simulink model "model_FS_PSH_IEEE39"  (R2020b)
settings: Solver=ode3  StartTime=0.0  StopTime=300  FixedStep=Ts  RelTol=1e-3
PostLoadFcn:
  | IEEE39BusLineLength;
  | vNomHV = 345E3;fNom=60;load('Dynamicload.mat');
InitFcn:
  | IEEE39BusLineLength;
  | vNomHV = 345E3;fNom=60;load('Dynamicload.mat');
values from neighbouring files (symbols this model uses):
  Rp = 0.05    [IEEE39BusLineLength.m]
  t_sw_off = 220    [MAIN_FS_PSH_IEEE39.m]    (also in MAIN_T_PSH_IEEE39.m; MAIN_VS_PSH.m = 45)
  t_sw_on = 130    [MAIN_FS_PSH_IEEE39.m]    (also in MAIN_T_PSH_IEEE39.m; MAIN_VS_PSH.m = 35)
  TL_10_11_len = 14    [IEEE39BusLineLength.m]
  TL_10_13_len = 14    [IEEE39BusLineLength.m]
  TL_13_14_len = 32    [IEEE39BusLineLength.m]
  TL_14_15_len = 70    [IEEE39BusLineLength.m]
  TL_15_16_len = 31.5    [IEEE39BusLineLength.m]
  TL_16_17_len = 26    [IEEE39BusLineLength.m]
  TL_16_19_len = 61    [IEEE39BusLineLength.m]
  TL_16_21_len = 46    [IEEE39BusLineLength.m]
  TL_16_24_len = 15    [IEEE39BusLineLength.m]
  TL_17_18_len = 26    [IEEE39BusLineLength.m]
  TL_17_27_len = 59    [IEEE39BusLineLength.m]
  TL_1_2_len = 134    [IEEE39BusLineLength.m]
  TL_1_39_len = 105    [IEEE39BusLineLength.m]
  TL_21_22_len = 47    [IEEE39BusLineLength.m]
  TL_22_23_len = 33    [IEEE39BusLineLength.m]
  TL_24_23_len = 88    [IEEE39BusLineLength.m]
  TL_25_26_len = 101    [IEEE39BusLineLength.m]
  TL_26_27_len = 46.5    [IEEE39BusLineLength.m]
  TL_26_28_len = 151    [IEEE39BusLineLength.m]
  TL_26_29_len = 200    [IEEE39BusLineLength.m]
  TL_28_29_len = 48    [IEEE39BusLineLength.m]
  TL_2_25_len = 28    [IEEE39BusLineLength.m]
  TL_2_2_len = 49    [IEEE39BusLineLength.m]
  TL_3_18_len = 42    [IEEE39BusLineLength.m]
  TL_3_4_len = 53    [IEEE39BusLineLength.m]
  TL_4_14_len = 33    [IEEE39BusLineLength.m]
  TL_4_5_len = 32.5    [IEEE39BusLineLength.m]
  TL_5_6_len = 14    [IEEE39BusLineLength.m]
  TL_5_8_len = 32    [IEEE39BusLineLength.m]
  TL_6_11_len = 26.5    [IEEE39BusLineLength.m]
  TL_6_7_len = 25.5    [IEEE39BusLineLength.m]
  TL_7_8_len = 15    [IEEE39BusLineLength.m]
  TL_8_9_len = 93    [IEEE39BusLineLength.m]
  TL_9_39_len = 136    [IEEE39BusLineLength.m]
  Ts = 25e-6    (= 2.5e-05)    [MAIN_FS_PSH_IEEE39.m]    (also in MAIN_T_PSH_IEEE39.m; MAIN_VS_PSH.m = 1e-07)
undefined symbols (not defined in the file or in its folder): D1, Delta, FS_PSH, load15, load16, load18, load20, load21, load23, load24, load25, load26, load27, load28, load29, load3, load39, load4, load7, load8
libraries: powerlib x216, sps_avr x10, powerlib_meascontrol x5, pid_lib x1
(part 5 of 8)

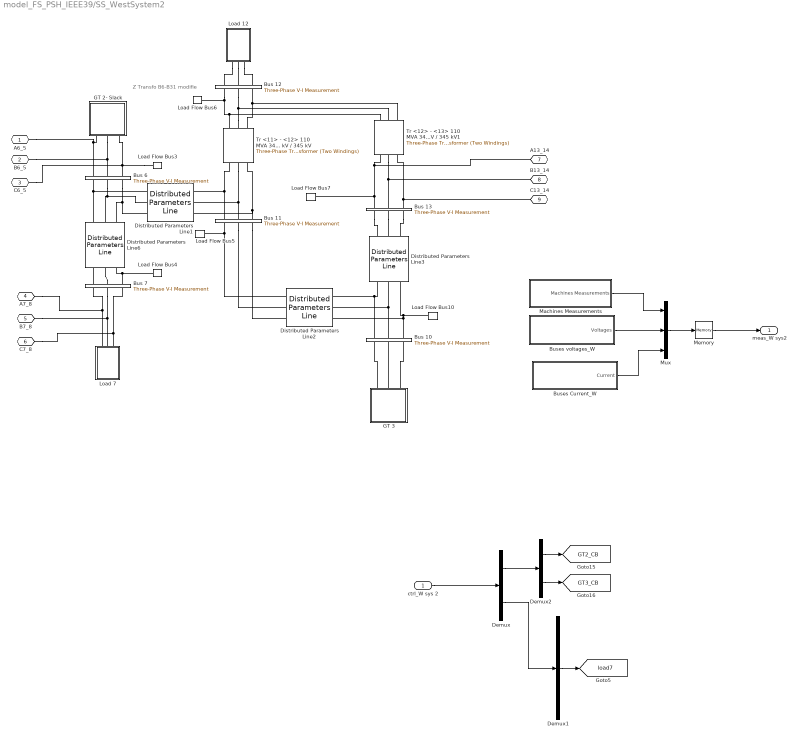
== system model_FS_PSH_IEEE39/SS_WestSystem2 ==
  note: Z Transfo B6-B31 modifie
  ctrl_W sys 2 : Inport
  Bus 10 : powerlib/Measurements/Three-Phase V-I Measurement  VoltageMeasurement=phase-to-ground  SetLabelV=on  LabelV=V_bus_10  Vpu=off  VpuLL=off  CurrentMeasurement=yes  SetLabelI=on  LabelI=I_bus_10  Ipu=off  Pbase=100e6  Vbase=230e3  OutputType=Complex  PhasorSimulation=off  PSBequivalent=0
  Bus 11 : powerlib/Measurements/Three-Phase V-I Measurement  VoltageMeasurement=phase-to-ground  SetLabelV=on  LabelV=V_bus_11  Vpu=off  VpuLL=off  CurrentMeasurement=yes  SetLabelI=on  LabelI=I_bus_11  Ipu=off  Pbase=100e6  Vbase=230e3  OutputType=Complex  PhasorSimulation=off  PSBequivalent=0
  Bus 12 : powerlib/Measurements/Three-Phase V-I Measurement  VoltageMeasurement=phase-to-ground  SetLabelV=on  LabelV=V_bus_12  Vpu=off  VpuLL=off  CurrentMeasurement=yes  SetLabelI=on  LabelI=I_bus_12  Ipu=off  Pbase=100e6  Vbase=230e3  OutputType=Complex  PhasorSimulation=off  PSBequivalent=0
  Bus 13 : powerlib/Measurements/Three-Phase V-I Measurement  VoltageMeasurement=phase-to-ground  SetLabelV=on  LabelV=V_bus_13  Vpu=off  VpuLL=off  CurrentMeasurement=yes  SetLabelI=on  LabelI=I_bus_13  Ipu=off  Pbase=100e6  Vbase=230e3  OutputType=Complex  PhasorSimulation=off  PSBequivalent=0
  Bus 6 : powerlib/Measurements/Three-Phase V-I Measurement  VoltageMeasurement=phase-to-ground  SetLabelV=on  LabelV=V_bus_6  Vpu=off  VpuLL=off  CurrentMeasurement=yes  SetLabelI=on  LabelI=I_bus_6  Ipu=off  Pbase=100e6  Vbase=230e3  OutputType=Complex  PhasorSimulation=off  PSBequivalent=0
  Bus 7 : powerlib/Measurements/Three-Phase V-I Measurement  VoltageMeasurement=phase-to-ground  SetLabelV=on  LabelV=V_bus_7  Vpu=off  VpuLL=off  CurrentMeasurement=yes  SetLabelI=on  LabelI=I_bus_7  Ipu=off  Pbase=100e6  Vbase=230e3  OutputType=Complex  PhasorSimulation=off  PSBequivalent=0
  Buses Current_W : Subsystem
  Buses voltages_W : Subsystem
  Demux : Demux  Outputs=[2 2]
  Demux1 : Demux  Outputs=[2 ]
  Demux2 : Demux  Outputs=2
  Distributed Parameters Line1 : powerlib/Elements/Distributed Parameters Line  Phases=3  Length=TL_6_11_len  Frequency=fNom  Resistance=[0.833 3.333]/TL_6_11_len  Inductance="[0.026  0.078]/TL_6_11_len"  Capacitance=[0.31e-6 0.141e-6]/TL_6_11_len  x1=[-0.000125 4.90236813149437e-09 0 0;-0.0001 4.73761402312569e-09 183127.021005182 -193527.239892428;-7.5e-05 4.57243909248611e-09 184942.800795633 -191792.737027805;-5e-05 4.40685801136803e-09 186742.152897159 -190041.198023314;-2.5e-05 4.2408854876405e-09 188524.917480904 -188272.778460778]  x2=[-0.000125 -1.4342554633322e-08 0 0;-0.0001 -1.44743326982834e-08 188556.811701446 -190108.544883478;-7.5e-05 -1.46048250693224e-08 190340.130987805 -188323.021034435;-5e-05 -1.47340201553523e-08 192106.543163165 -186520.769245761;-2.5e-05 -1.48619064805184e-08 193855.891324581 -184701.949603881]  x3=[-0.000125 -1.81011006279439e-10 0 0;-0.0001 -1.87198811943795e-10 1012.19433406295 -1197.40014896563;-7.5e-05 -1.93369989527271e-10 1023.43451008816 -1187.80734434082;-5e-05 -1.99523990870192e-10 1034.58377874259 -1178.10903179967;-2.5e-05 -2.05660269338577e-10 1045.64114968372 -1168.30607280236]  x4=[-0.000125 1.68385779335451e-10 0 0;-0.0001 1.74132809904858e-10 246.070217535326 -146.122053826147;-7.5e-05 1.79864372991236e-10 247.436293615228 -143.796492599063;-5e-05 1.85579959484012e-10 248.780390972829 -141.45815853606;-2.5e-05 1.91279061691744e-10 250.102390217632 -139.107259341491]  x5=0.000104871349757691  V1=ones(3,3)  V2=ones(3,3)  I1=ones(3,3)  I2=ones(3,3)  nHarmo=1  Measurements=None  Decoupling=off  VsMag0=0  VrMag0=0  VsAngle0=0  VrAngle0=0  IsMag0=0  IrMag0=0  IsAngle0=0  IrAngle0=0
  Distributed Parameters Line2 : powerlib/Elements/Distributed Parameters Line  Phases=3  Length=TL_10_11_len  Frequency=fNom  Resistance=[0.476 1.904]/TL_10_11_len  Inductance="[0.014  0.04]/TL_10_11_len"  Capacitance=[0.162e-6 0.074e-6]/TL_10_11_len  x1=[-7.5e-05 -1.46049279170452e-08 0 0;-5e-05 -1.47340887255765e-08 192106.543163165 -186520.769245761;-2.5e-05 -1.48619407671533e-08 193855.891324581 -184701.949603881]  x2=[-7.5e-05 -2.31631319093915e-08 0 0;-5e-05 -2.32876424160693e-08 195466.101592622 -184887.987151561;-2.5e-05 -2.34100843796963e-08 197199.912483554 -183037.577926856]  x3=[-7.5e-05 -1.20973818921581e-10 0 0;-5e-05 -1.26341409378821e-10 1010.52803842152 -1242.83594676881;-2.5e-05 -1.31697777461561e-10 1022.19650500434 -1233.25683348948]  x4=[-7.5e-05 7.40590073052612e-11 0 0;-5e-05 7.90894066759697e-11 294.937649217573 -30.8703627073713;-2.5e-05 8.41127808682744e-11 295.215353287942 -28.08936050336]  x5=5.44058820349418e-05  V1=ones(3,3)  V2=ones(3,3)  I1=ones(3,3)  I2=ones(3,3)  nHarmo=1  Measurements=None  Decoupling=off  VsMag0=0  VrMag0=0  VsAngle0=0  VrAngle0=0  IsMag0=0  IrMag0=0  IsAngle0=0  IrAngle0=0
  Distributed Parameters Line3 : powerlib/Elements/Distributed Parameters Line  Phases=3  Length=TL_10_13_len  Frequency=fNom  Resistance=[0.476 1.904]/TL_10_13_len  Inductance=[0.014 0.04]/TL_10_13_len  Capacitance=[0.162e-6 0.074e-6]/TL_10_13_len  x1=[-7.5e-05 -1.85919269091365e-08 0 0;-5e-05 -1.87360708053477e-08 257967.853677424 -71921.0706051768;-2.5e-05 -1.88785504554162e-08 257278.56069942 -74349.1214410131]  x2=[-7.5e-05 -2.31631319093915e-08 0 0;-5e-05 -2.32876424160693e-08 257850.744524134 -76834.6159821403;-2.5e-05 -2.34100843796963e-08 257115.148573608 -79261.3448713978]  x3=[-7.5e-05 -1.9729013706856e-10 0 0;-5e-05 -2.00122610987713e-10 1799.42783654337 -341.693872198189;-2.5e-05 -2.02937308859429e-10 1796.12756372396 -358.637663817273]  x4=[-7.5e-05 1.41714968743232e-10 0 0;-5e-05 1.44134764486409e-10 -42.3684337823979 -147.97249719393;-2.5e-05 1.46541757346403e-10 -43.7611636427956 -147.566548222069]  x5=5.44058820349418e-05  V1=ones(3,3)  V2=ones(3,3)  I1=ones(3,3)  I2=ones(3,3)  nHarmo=1  Measurements=None  Decoupling=off  VsMag0=0  VrMag0=0  VsAngle0=0  VrAngle0=0  IsMag0=0  IrMag0=0  IsAngle0=0  IrAngle0=0
  Distributed Parameters Line6 : powerlib/Elements/Distributed Parameters Line  Phases=3  Length=TL_6_7_len  Frequency=fNom  Resistance=[0.714 2.857]/TL_6_7_len  Inductance=[0.029 0.087]/TL_6_7_len  Capacitance=[0.252e-6 0.114e-6]/TL_6_7_len  x1=[-0.0001 4.73761402312569e-09 259163.016573719 -61829.0323636399;-7.5e-05 4.57243909248611e-09 258568.782925244 -64268.7952221604;-5e-05 4.40685801136803e-09 257951.581702399 -66702.8493546806;-2.5e-05 4.2408854876405e-09 257311.467728565 -69130.9785544385]  x2=[-0.0001 4.12646376630165e-09 259289.948818673 -48646.1844692721;-7.5e-05 3.96483863419745e-09 258819.953112779 -51087.7289997077;-5e-05 3.80286132220067e-09 258326.967522127 -53524.7356226591;-2.5e-05 3.64054621807272e-09 257811.035836546 -55956.9878691072]  x3=[-0.0001 -8.28425316453442e-12 -433.188488031618 -79.7957266342144;-7.5e-05 -8.62804148707643e-12 -433.921305740028 -75.7095112058845;-5e-05 -8.97106341708535e-12 -434.615580049085 -71.6165708210094;-2.5e-05 -9.31328848536999e-12 -435.271249289331 -67.5172690382197]  x4=[-0.0001 1.51239119220935e-11 1964.32766038478 -220.748781181744;-7.5e-05 1.5097572753948e-11 1962.15991096584 -239.252028488418;-5e-05 1.50698925320947e-11 1959.8178711582 -257.734024046541;-2.5e-05 1.50408737152511e-11 1957.30174899538 -276.193126178405]  x5=9.9589156036187e-05  V1=ones(3,3)  V2=ones(3,3)  I1=ones(3,3)  I2=ones(3,3)  nHarmo=1  Measurements=None  Decoupling=off  VsMag0=0  VrMag0=0  VsAngle0=0  VrAngle0=0  IsMag0=0  IrMag0=0  IsAngle0=0  IrAngle0=0
  GT 2- Slack : Subsystem
  GT 3 : Subsystem
  Load 12 : Subsystem
  Load 7 : Subsystem
  Load Flow Bus10 : powerlib/Measurements/Load Flow Bus  LConnTagsString=a  Phases=single  Connectors=on one side  ID=Bus-10  Vbase=345e+003  Vref=1  Vangle=0  VLF=1.011  VLFb=1  VLFc=1  angleLF=22.22  angleLFb=0  angleLFc=0
      settings: AttributesFormatString=%<ID>\n%<Vbase>V\n%<VLF>pu\n%<angleLF>deg.
  Load Flow Bus3 : powerlib/Measurements/Load Flow Bus  LConnTagsString=a  Phases=single  Connectors=on one side  ID=Bus-6  Vbase=345e+003  Vref=1  Vangle=0  VLF=1.003  VLFb=1  VLFc=1  angleLF=20.92  angleLFb=0  angleLFc=0
      settings: AttributesFormatString=%<ID>\n%<Vbase>V\n%<VLF>pu\n%<angleLF>deg.
  Load Flow Bus4 : powerlib/Measurements/Load Flow Bus  LConnTagsString=a  Phases=single  Connectors=on one side  ID=Bus-7  Vbase=345e+003  Vref=1  Vangle=0  VLF=0.9928  VLFb=1  VLFc=1  angleLF=19.19  angleLFb=0  angleLFc=0
      settings: AttributesFormatString=%<ID>\n%<Vbase>V\n%<VLF>pu\n%<angleLF>deg.
  Load Flow Bus5 : powerlib/Measurements/Load Flow Bus  LConnTagsString=a  Phases=single  Connectors=on one side  ID=Bus-11  Vbase=345e+003  Vref=1  Vangle=0  VLF=1.007  VLFb=1  VLFc=1  angleLF=21.76  angleLFb=0  angleLFc=0
      settings: AttributesFormatString=%<ID>\n%<Vbase>V\n%<VLF>pu\n%<angleLF>deg.
  Load Flow Bus6 : powerlib/Measurements/Load Flow Bus  LConnTagsString=a  Phases=single  Connectors=on one side  ID=Bus-12  Vbase=345e+003  Vref=1  Vangle=0  VLF=0.996  VLFb=1  VLFc=1  angleLF=51.6  angleLFb=0  angleLFc=0
      settings: AttributesFormatString=%<ID>\n%<Vbase>V\n%<VLF>pu\n%<angleLF>deg.
  Load Flow Bus7 : powerlib/Measurements/Load Flow Bus  LConnTagsString=a  Phases=single  Connectors=on one side  ID=Bus-13  Vbase=345e+003  Vref=1  Vangle=0  VLF=1.007  VLFb=1  VLFc=1  angleLF=21.59  angleLFb=0  angleLFc=0
      settings: AttributesFormatString=%<ID>\n%<Vbase>V\n%<VLF>pu\n%<angleLF>deg.
  Machines Measurements : Subsystem
      mask Display: disp('Machines Measurements')
  Memory : Memory
  Mux : Mux  Inputs=3
  Tr <11> - <12> 110 MVA 345 kV / 345 kV : powerlib/Elements/Three-Phase Transformer (Two Windings)  Winding1Connection=Delta (D1)  Winding2Connection=Yg  CoreType=Three single-phase transformers  SetSaturation=off  Hysteresis=off  DataFile='hysteresis'  SetInitialFlux=off  Measurements=None  UNITS=pu  NominalPower=[ 110e6 fNom]  Winding1="[345e3 0.0016*110/100/2   0.0435*110/100/2]"  Winding2="[ 1.006*345e3 0.0016*110/100/2   0.0435*110/100/2]"  Rm=500  Lm=500  L0=0.5  Saturation="[ 0,0  ;  0.005,1.2  ;  1.0,1.4 ]"  InitialFluxes=[ 0.8 , -0.8 , 0.7 ]  BreakLoop=off  DiscreteSolver=Trapezoidal iterative  DataType=off  TransfoNumber=0
  Tr <12> - <13> 110 MVA 345 kV / 345 kV1 : powerlib/Elements/Three-Phase Transformer (Two Windings)  Winding1Connection=Delta (D1)  Winding2Connection=Yg  CoreType=Three single-phase transformers  SetSaturation=off  Hysteresis=off  DataFile='hysteresis'  SetInitialFlux=off  Measurements=None  UNITS=pu  NominalPower=[ 110e6 fNom]  Winding1="[ 345e3  0.0016*110/100/2   0.0435*110/100/2]"  Winding2="[ 1.006*345e3  0.0016*110/100/2   0.0435*110/100/2]"  Rm=500  Lm=500  L0=0.5  Saturation="[ 0,0  ;  0.005,1.2  ;  1.0,1.4 ]"  InitialFluxes=[ 0.8 , -0.8 , 0.7 ]  BreakLoop=off  DiscreteSolver=Trapezoidal iterative  DataType=off  TransfoNumber=0
  A6_5 : PMIOPort  Side=Left
  B6_5 : PMIOPort  Port=2  Side=Left
  C6_5 : PMIOPort  Port=3  Side=Left
  A7_8 : PMIOPort  Port=4  Side=Left
  B7_8 : PMIOPort  Port=5  Side=Left
  C7_8 : PMIOPort  Port=6  Side=Left
  A13_14 : PMIOPort  Port=7  Side=Right
  B13_14 : PMIOPort  Port=8  Side=Right
  C13_14 : PMIOPort  Port=9  Side=Right
  meas_W sys2 : Outport
  tag scope: GT2_CB=global, GT3_CB=global, load7=global
  wires:
  Mux/1 -> Memory/1
  Memory/1 -> meas_W sys2/1
  Buses voltages_W/1(Voltages) -> Mux/2
  Machines Measurements/1(Machines Measurements) -> Mux/1
  Buses Current_W/1(Current) -> Mux/3
  ctrl_W sys 2/1 -> Demux/1
  Demux/2 -> Demux1/1
  Demux/1 -> Demux2/1
  Demux2/1 -> [GT2_CB]
  Demux2/2 -> [GT3_CB]
  Demux1/1 -> [load7]
  connections:
  Bus 7/RConn3 -- Distributed Parameters Line6/RConn1 -- Load Flow Bus4/LConn1
  Load Flow Bus3/LConn1 -- C6_5/RConn1 -- GT 2- Slack/RConn3 -- Bus 6/RConn3
  GT 2- Slack/RConn2 -- B6_5/RConn1 -- Bus 6/RConn2
  GT 2- Slack/RConn1 -- Bus 6/RConn1 -- A6_5/RConn1
  Bus 6/LConn3 -- Distributed Parameters Line1/LConn3 -- Distributed Parameters Line6/LConn1
  Bus 6/LConn2 -- Distributed Parameters Line1/LConn2 -- Distributed Parameters Line6/LConn2
  Bus 6/LConn1 -- Distributed Parameters Line1/LConn1 -- Distributed Parameters Line6/LConn3
  Bus 13/RConn3 -- Tr <12> - <13> 110 MVA 345 kV / 345 kV1/LConn3 -- C13_14/RConn1
  Tr <12> - <13> 110 MVA 345 kV / 345 kV1/LConn2 -- Bus 13/RConn2 -- B13_14/RConn1
  Load Flow Bus7/LConn1 -- Bus 13/RConn1 -- Tr <12> - <13> 110 MVA 345 kV / 345 kV1/LConn1 -- A13_14/RConn1
  Load 12/LConn3 -- Bus 12/RConn3
  Load 12/LConn2 -- Bus 12/RConn2
  Load 12/LConn1 -- Bus 12/RConn1
  Bus 12/LConn3 -- Tr <11> - <12> 110 MVA 345 kV / 345 kV/RConn3 -- Tr <12> - <13> 110 MVA 345 kV / 345 kV1/RConn3
  Tr <11> - <12> 110 MVA 345 kV / 345 kV/RConn2 -- Bus 12/LConn2 -- Tr <12> - <13> 110 MVA 345 kV / 345 kV1/RConn2
  Load Flow Bus6/LConn1 -- Tr <12> - <13> 110 MVA 345 kV / 345 kV1/RConn1 -- Tr <11> - <12> 110 MVA 345 kV / 345 kV/RConn1 -- Bus 12/LConn1
  Bus 11/RConn3 -- Tr <11> - <12> 110 MVA 345 kV / 345 kV/LConn3 -- Distributed Parameters Line1/RConn3
  Tr <11> - <12> 110 MVA 345 kV / 345 kV/LConn2 -- Distributed Parameters Line1/RConn2 -- Bus 11/RConn2
  Tr <11> - <12> 110 MVA 345 kV / 345 kV/LConn1 -- Bus 11/RConn1 -- Distributed Parameters Line1/RConn1
  Bus 11/LConn3 -- Distributed Parameters Line2/LConn3
  Bus 11/LConn2 -- Distributed Parameters Line2/LConn2
  Load Flow Bus5/LConn1 -- Distributed Parameters Line2/LConn1 -- Bus 11/LConn1
  Bus 10/RConn3 -- Distributed Parameters Line2/RConn3 -- Distributed Parameters Line3/RConn1 -- Load Flow Bus10/LConn1
  Distributed Parameters Line2/RConn2 -- Distributed Parameters Line3/RConn2 -- Bus 10/RConn2
  Bus 10/RConn1 -- Distributed Parameters Line3/RConn3 -- Distributed Parameters Line2/RConn1
  GT 3/RConn3 -- Bus 10/LConn3
  GT 3/RConn2 -- Bus 10/LConn2
  GT 3/RConn1 -- Bus 10/LConn1
  Bus 7/LConn1 -- A7_8/RConn1 -- Load 7/LConn1
  Bus 7/LConn2 -- Load 7/LConn2 -- B7_8/RConn1
  Bus 7/LConn3 -- C7_8/RConn1 -- Load 7/LConn3
  Distributed Parameters Line6/RConn2 -- Bus 7/RConn2
  Bus 7/RConn1 -- Distributed Parameters Line6/RConn3
  Bus 13/LConn1 -- Distributed Parameters Line3/LConn3
  Bus 13/LConn2 -- Distributed Parameters Line3/LConn2
  Bus 13/LConn3 -- Distributed Parameters Line3/LConn1

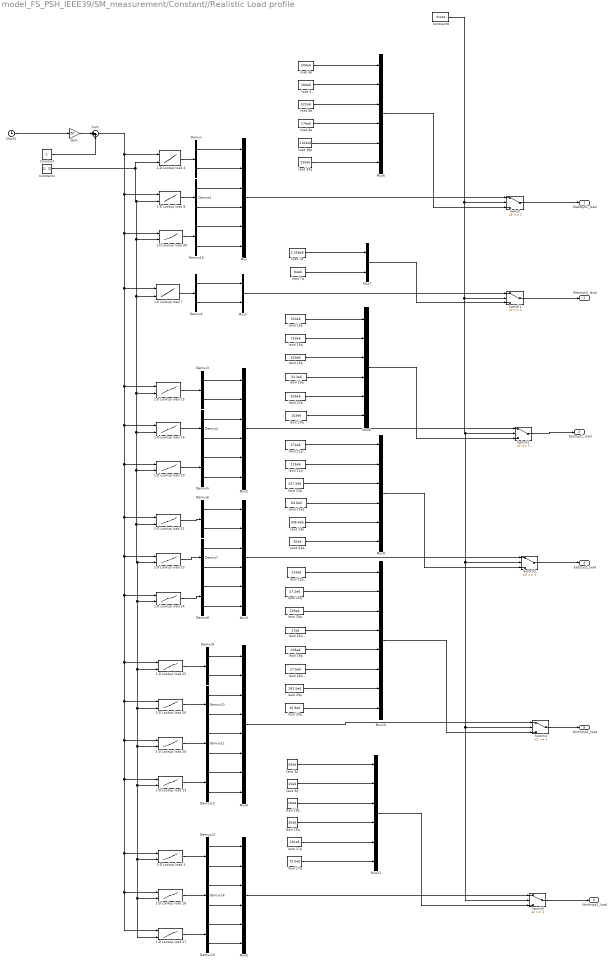
== system model_FS_PSH_IEEE39/SM_measurement/Constant//Realistic Load profile ==
  1-D Lookup load 15 : Lookup_n-D  BreakpointsForDimension1=[1:18000]  BreakpointsForDimension2=[1 2]  Table=load15  InterpMethod=Flat  ExtrapMethod=Cubic spline  DiagnosticForOutOfRangeInput=Error  InternalRulePriority=Speed  RndMeth=Simplest  InputSameDT=on
      settings: InputPortMap=u0,u1
  1-D Lookup load 16 : Lookup_n-D  BreakpointsForDimension1=[1:18000]  BreakpointsForDimension2=[1 2]  Table=load16  InterpMethod=Flat  ExtrapMethod=Cubic spline  DiagnosticForOutOfRangeInput=Error  InternalRulePriority=Speed  RndMeth=Simplest  InputSameDT=on
      settings: InputPortMap=u0,u1
  1-D Lookup load 18 : Lookup_n-D  BreakpointsForDimension1=[1:18000]  BreakpointsForDimension2=[1 2]  Table=load18  InterpMethod=Flat  ExtrapMethod=Cubic spline  DiagnosticForOutOfRangeInput=Error  InternalRulePriority=Speed  RndMeth=Simplest  InputSameDT=on
      settings: InputPortMap=u0,u1
  1-D Lookup load 20 : Lookup_n-D  BreakpointsForDimension1=[1:18000]  BreakpointsForDimension2=[1 2]  Table=load20  InterpMethod=Flat  ExtrapMethod=Cubic spline  DiagnosticForOutOfRangeInput=Error  InternalRulePriority=Speed  RndMeth=Simplest  InputSameDT=on
      settings: InputPortMap=u0,u1
  1-D Lookup load 21 : Lookup_n-D  BreakpointsForDimension1=[1:18000]  BreakpointsForDimension2=[1 2]  Table=load21  InterpMethod=Flat  ExtrapMethod=Cubic spline  DiagnosticForOutOfRangeInput=Error  InternalRulePriority=Speed  RndMeth=Simplest  InputSameDT=on
      settings: InputPortMap=u0,u1
  1-D Lookup load 23 : Lookup_n-D  BreakpointsForDimension1=[1:18000]  BreakpointsForDimension2=[1 2]  Table=load23  InterpMethod=Flat  ExtrapMethod=Cubic spline  DiagnosticForOutOfRangeInput=Error  InternalRulePriority=Speed  RndMeth=Simplest  InputSameDT=on
      settings: InputPortMap=u0,u1
  1-D Lookup load 24 : Lookup_n-D  BreakpointsForDimension1=[1:18000]  BreakpointsForDimension2=[1 2]  Table=load24  InterpMethod=Flat  ExtrapMethod=Cubic spline  DiagnosticForOutOfRangeInput=Error  InternalRulePriority=Speed  RndMeth=Simplest  InputSameDT=on
      settings: InputPortMap=u0,u1
  1-D Lookup load 25 : Lookup_n-D  BreakpointsForDimension1=[1:18000]  BreakpointsForDimension2=[1 2]  Table=load25  InterpMethod=Flat  ExtrapMethod=Cubic spline  DiagnosticForOutOfRangeInput=Error  InternalRulePriority=Speed  RndMeth=Simplest  InputSameDT=on
      settings: InputPortMap=u0,u1
  1-D Lookup load 26 : Lookup_n-D  BreakpointsForDimension1=[1:18000]  BreakpointsForDimension2=[1 2]  Table=load26  InterpMethod=Flat  ExtrapMethod=Cubic spline  DiagnosticForOutOfRangeInput=Error  InternalRulePriority=Speed  RndMeth=Simplest  InputSameDT=on
      settings: InputPortMap=u0,u1
  1-D Lookup load 27 : Lookup_n-D  BreakpointsForDimension1=[1:18000]  BreakpointsForDimension2=[1 2]  Table=load27  InterpMethod=Flat  ExtrapMethod=Cubic spline  DiagnosticForOutOfRangeInput=Error  InternalRulePriority=Speed  RndMeth=Simplest  InputSameDT=on
      settings: InputPortMap=u0,u1
  1-D Lookup load 28 : Lookup_n-D  BreakpointsForDimension1=[1:18000]  BreakpointsForDimension2=[1 2]  Table=load28  InterpMethod=Flat  ExtrapMethod=Cubic spline  DiagnosticForOutOfRangeInput=Error  InternalRulePriority=Speed  RndMeth=Simplest  InputSameDT=on
      settings: InputPortMap=u0,u1
  1-D Lookup load 29 : Lookup_n-D  BreakpointsForDimension1=[1:18000]  BreakpointsForDimension2=[1 2]  Table=load29  InterpMethod=Flat  ExtrapMethod=Cubic spline  DiagnosticForOutOfRangeInput=Error  InternalRulePriority=Speed  RndMeth=Simplest  InputSameDT=on
      settings: InputPortMap=u0,u1
  1-D Lookup load 3 : Lookup_n-D  BreakpointsForDimension1=[1:18000]  BreakpointsForDimension2=[1 2]  Table=load3  InterpMethod=Flat  ExtrapMethod=Cubic spline  DiagnosticForOutOfRangeInput=Error  InternalRulePriority=Speed  RndMeth=Simplest  InputSameDT=on
      settings: InputPortMap=u0,u1
  1-D Lookup load 39 : Lookup_n-D  BreakpointsForDimension1=[1:18000]  BreakpointsForDimension2=[1 2]  Table=load39  InterpMethod=Flat  ExtrapMethod=Cubic spline  DiagnosticForOutOfRangeInput=Error  InternalRulePriority=Speed  RndMeth=Simplest  InputSameDT=on
      settings: InputPortMap=u0,u1
  1-D Lookup load 4 : Lookup_n-D  BreakpointsForDimension1=[1:18000]  BreakpointsForDimension2=[1 2]  Table=load4  InterpMethod=Flat  ExtrapMethod=Cubic spline  DiagnosticForOutOfRangeInput=Error  InternalRulePriority=Speed  RndMeth=Simplest  InputSameDT=on
      settings: InputPortMap=u0,u1
  1-D Lookup load 7 : Lookup_n-D  BreakpointsForDimension1=[1:18000]  BreakpointsForDimension2=[1 2]  Table=load7  InterpMethod=Flat  ExtrapMethod=Cubic spline  DiagnosticForOutOfRangeInput=Error  InternalRulePriority=Speed  RndMeth=Simplest  InputSameDT=on
      settings: InputPortMap=u0,u1
  1-D Lookup load 8 : Lookup_n-D  BreakpointsForDimension1=[1:18000]  BreakpointsForDimension2=[1 2]  Table=load8  InterpMethod=Flat  ExtrapMethod=Cubic spline  DiagnosticForOutOfRangeInput=Error  InternalRulePriority=Speed  RndMeth=Simplest  InputSameDT=on
      settings: InputPortMap=u0,u1
  Clock1 : Clock
  Constant : Constant  SampleTime=20e-3
  Constant1 : Constant  Value="[1  2]"  VectorParams1D=off  SampleTime=20e-3
  Constant6 : Constant  Value=mode
  Demux{,1..16} (17 alike) : Demux  Outputs=2
  Gain : Gain  Gain=50
  Mux{,2..3,5..6,8..9,11} (8 alike) : Mux  Inputs=6
  Mux1 : Mux  Inputs=2
  Mux10 : Mux  Inputs=8
  Mux4 : Mux  Inputs=8
  Mux7 : Mux  Inputs=2
  Sum : Sum  Inputs=|++
  Switch{,1..5} (6 alike) : Switch  Threshold=1
  laod 15p : Constant  Value=320e6  VectorParams1D=off  SampleTime=20e-3
  laod 15q : Constant  Value=153e6  VectorParams1D=off  SampleTime=20e-3
  laod 16p : Constant  Value=329e6  VectorParams1D=off  SampleTime=20e-3
  laod 16q : Constant  Value=32.3e6  VectorParams1D=off  SampleTime=20e-3
  laod 18p : Constant  Value=158e6  VectorParams1D=off  SampleTime=20e-3
  laod 18q : Constant  Value=30e6  VectorParams1D=off  SampleTime=20e-3
  laod 20p : Constant  Value=628e6  VectorParams1D=off  SampleTime=20e-3
  laod 20q : Constant  Value=103e6  VectorParams1D=off  SampleTime=20e-3
  laod 21p : Constant  Value=274e6  VectorParams1D=off  SampleTime=20e-3
  laod 21q : Constant  Value=115e6  VectorParams1D=off  SampleTime=20e-3
  laod 23p : Constant  Value=247.5e6  VectorParams1D=off  SampleTime=20e-3
  laod 23p1 : Constant  Value=84.6e6  VectorParams1D=off  SampleTime=20e-3
  laod 24p : Constant  Value=308.6e6  SampleTime=20e-3
  laod 24q : Constant  Value=-92e6  VectorParams1D=off  SampleTime=20e-3
  laod 25p : Constant  Value=224e6  VectorParams1D=off  SampleTime=20e-3
  laod 25q : Constant  Value=47.2e6  VectorParams1D=off  SampleTime=20e-3
  laod 26p : Constant  Value=139e6  VectorParams1D=off  SampleTime=20e-3
  laod 26q : Constant  Value=17e6  VectorParams1D=off  SampleTime=20e-3
  laod 27p : Constant  Value=281e6  VectorParams1D=off  SampleTime=20e-3
  laod 27q : Constant  Value=75.5e6  VectorParams1D=off  SampleTime=20e-3
  laod 28p : Constant  Value=206e6  VectorParams1D=off  SampleTime=20e-3
  laod 28q : Constant  Value=27.6e6  VectorParams1D=off  SampleTime=20e-3
  laod 29p : Constant  Value=283.5e6  VectorParams1D=off  SampleTime=20e-3
  laod 29q : Constant  Value=26.9e6  VectorParams1D=off  SampleTime=20e-3
  laod 3p : Constant  Value=50e6  VectorParams1D=off  SampleTime=20e-3
  laod 3q : Constant  Value=25e6  VectorParams1D=off  SampleTime=20e-3
  load 39p : Constant  Value=1104e6  VectorParams1D=off  SampleTime=20e-3
  load 39q : Constant  Value=250e6  VectorParams1D=off  SampleTime=20e-3
  load 4 : Constant  Value=184e6  VectorParams1D=off  SampleTime=20e-3
  load 4p : Constant  Value=500e6  VectorParams1D=off  SampleTime=20e-3
  load 7p : Constant  Value=2.338e8  VectorParams1D=off  SampleTime=20e-3
  load 7q : Constant  Value=84e6  VectorParams1D=off  SampleTime=20e-3
  load 8p : Constant  Value=522e6  VectorParams1D=off  SampleTime=20e-3
  load 8q : Constant  Value=176e6  VectorParams1D=off  SampleTime=20e-3
  Westsys1_load : Outport
  Westsys2_laod : Outport  Port=2
  Eastsys1_load : Outport  Port=3
  Eastsys2_load : Outport  Port=4
  Northsys1_load : Outport  Port=5
  Northsys2_load : Outport  Port=6
  wires:
  Mux2/1 -> Switch2/1
  Constant/1 -> Sum/2
  Mux/1 -> Switch/1
  Mux1/1 -> Switch1/1
  Mux5/1 -> Switch5/1
  1-D Lookup load 15/1 -> Demux3/1
  Demux2/2 -> Mux1/2
  Demux5/2 -> Mux2/6
  Demux7/2 -> Mux3/4
  Demux10/2 -> Mux4/4
  Sum/1 -> 1-D Lookup load 28/1, 1-D Lookup load 27/1, 1-D Lookup load 18/1, 1-D Lookup load 3/1, 1-D Lookup load 29/1, 1-D Lookup load 26/1, 1-D Lookup load 25/1, 1-D Lookup load 24/1, 1-D Lookup load 23/1, 1-D Lookup load 21/1, 1-D Lookup load 20/1, 1-D Lookup load 16/1, 1-D Lookup load 15/1, 1-D Lookup load 7/1, 1-D Lookup load 39/1, 1-D Lookup load 8/1, 1-D Lookup load 4/1
  1-D Lookup load 4/1 -> Demux/1
  Demux/1 -> Mux/1
  Demux/2 -> Mux/2
  1-D Lookup load 8/1 -> Demux1/1
  Demux1/1 -> Mux/3
  Demux1/2 -> Mux/4
  Demux16/1 -> Mux/5
  Demux16/2 -> Mux/6
  1-D Lookup load 39/1 -> Demux16/1
  1-D Lookup load 7/1 -> Demux2/1
  Demux2/1 -> Mux1/1
  Demux3/1 -> Mux2/1
  Demux3/2 -> Mux2/2
  1-D Lookup load 16/1 -> Demux4/1
  Demux4/1 -> Mux2/3
  Demux4/2 -> Mux2/4
  Demux5/1 -> Mux2/5
  1-D Lookup load 20/1 -> Demux5/1
  Demux6/2 -> Mux3/2
  Demux6/1 -> Mux3/1
  1-D Lookup load 21/1 -> Demux6/1
  Demux7/1 -> Mux3/3
  1-D Lookup load 23/1 -> Demux7/1
  1-D Lookup load 24/1 -> Demux8/1
  Demux8/1 -> Mux3/5
  Demux8/2 -> Mux3/6
  Demux9/2 -> Mux4/2
  Demux9/1 -> Mux4/1
  1-D Lookup load 25/1 -> Demux9/1
  1-D Lookup load 26/1 -> Demux10/1
  Demux10/1 -> Mux4/3
  Demux11/1 -> Mux4/5
  Demux11/2 -> Mux4/6
  1-D Lookup load 28/1 -> Demux11/1
  Demux12/1 -> Mux4/7
  Demux12/2 -> Mux4/8
  1-D Lookup load 29/1 -> Demux12/1
  1-D Lookup load 3/1 -> Demux13/1
  Demux13/1 -> Mux5/1
  Demux13/2 -> Mux5/2
  Constant1/1 -> 1-D Lookup load 7/2, 1-D Lookup load 20/2, 1-D Lookup load 27/2, 1-D Lookup load 18/2, 1-D Lookup load 3/2, 1-D Lookup load 29/2, 1-D Lookup load 28/2, 1-D Lookup load 26/2, 1-D Lookup load 25/2, 1-D Lookup load 24/2, 1-D Lookup load 23/2, 1-D Lookup load 21/2, 1-D Lookup load 16/2, 1-D Lookup load 15/2, 1-D Lookup load 39/2, 1-D Lookup load 8/2, 1-D Lookup load 4/2
  Demux14/1 -> Mux5/3
  Demux14/2 -> Mux5/4
  1-D Lookup load 18/1 -> Demux14/1
  Demux15/1 -> Mux5/5
  Demux15/2 -> Mux5/6
  1-D Lookup load 27/1 -> Demux15/1
  Clock1/1 -> Gain/1
  Gain/1 -> Sum/1
  Mux6/1 -> Switch/3
  load 4p/1 -> Mux6/1
  load 4/1 -> Mux6/2
  load 8p/1 -> Mux6/3
  load 8q/1 -> Mux6/4
  load 39p/1 -> Mux6/5
  load 39q/1 -> Mux6/6
  Constant6/1 -> Switch5/2, Switch4/2, Switch3/2, Switch2/2, Switch1/2, Switch/2
  Switch/1 -> Westsys1_load/1
  Mux7/1 -> Switch1/3
  load 7q/1 -> Mux7/2
  load 7p/1 -> Mux7/1
  Switch1/1 -> Westsys2_laod/1
  Switch2/1 -> Eastsys1_load/1
  laod 20q/1 -> Mux8/6
  laod 15p/1 -> Mux8/1
  laod 15q/1 -> Mux8/2
  laod 16p/1 -> Mux8/3
  laod 16q/1 -> Mux8/4
  laod 20p/1 -> Mux8/5
  Mux8/1 -> Switch2/3
  Switch3/1 -> Eastsys2_load/1
  Mux3/1 -> Switch3/1
  laod 23p1/1 -> Mux9/4
  laod 21q/1 -> Mux9/2
  laod 21p/1 -> Mux9/1
  laod 23p/1 -> Mux9/3
  laod 24p/1 -> Mux9/5
  laod 24q/1 -> Mux9/6
  Mux9/1 -> Switch3/3
  Mux10/1 -> Switch4/3
  laod 26q/1 -> Mux10/4
  laod 25q/1 -> Mux10/2
  laod 25p/1 -> Mux10/1
  laod 26p/1 -> Mux10/3
  laod 28p/1 -> Mux10/5
  laod 28q/1 -> Mux10/6
  laod 29p/1 -> Mux10/7
  laod 29q/1 -> Mux10/8
  Switch4/1 -> Northsys1_load/1
  Mux4/1 -> Switch4/1
  Mux11/1 -> Switch5/3
  laod 3p/1 -> Mux11/1
  laod 3q/1 -> Mux11/2
  laod 18p/1 -> Mux11/3
  laod 18q/1 -> Mux11/4
  laod 27p/1 -> Mux11/5
  laod 27q/1 -> Mux11/6
  Switch5/1 -> Northsys2_load/1

== system model_FS_PSH_IEEE39/SM_measurement/GT control ==
  note: 10
  note: 9
  note: 8
  note: 7
  note: 6
  note: 5
  note: 4
  note: 3
  note: 2
  note: 1
  Bus Creator : BusCreator  Inputs=3
  Constant{1..6,8,10,12,14} (10 alike) : Constant
  Mux1 : Mux  Inputs=3
  Mux2 : Mux
  Mux6 : Mux  Inputs=3
  GT_CBs_ctrl : Outport
  wires:
  Constant1/1 -> Mux1/2
  Constant10/1 -> Mux1/1
  Constant12/1 -> Mux2/4
  Constant5/1 -> Mux2/3
  Constant2/1 -> Mux2/2
  Constant3/1 -> Mux2/1
  Constant4/1 -> Mux6/3
  Constant8/1 -> Mux6/2
  Constant14/1 -> Mux1/3
  Constant6/1 -> Mux6/1
  Bus Creator/1 -> GT_CBs_ctrl/1
  Mux2/1 -> Bus Creator/2  "Eastsystem GT ctrl"
  Mux6/1 -> Bus Creator/1  "Westsystem GT ctrl"
  Mux1/1 -> Bus Creator/3  "Northsystem GT ctrl"

== system model_FS_PSH_IEEE39/SS_EastSystem1/Buses current_E ==
  Mux3 : Mux  Inputs=5
  current : Outport
  wires:
  Mux3/1 -> current/1
  [I_bus_14] -> Mux3/1
  [I_L15] -> Mux3/2
  [I_L16] -> Mux3/3
  [I_bus_19] -> Mux3/4
  [I_L20] -> Mux3/5

== system model_FS_PSH_IEEE39/SS_EastSystem1/Buses voltages_E ==
  Mux3 : Mux  Inputs=5
  Voltages : Outport
  wires:
  [V_L20] -> Mux3/5
  [V_bus_19] -> Mux3/4
  [V_L16] -> Mux3/3
  [V_L15] -> Mux3/2
  [V_bus_14] -> Mux3/1
  Mux3/1 -> Voltages/1

== system model_FS_PSH_IEEE39/SS_EastSystem1/GT 4 ==
  5 MW : powerlib/Elements/Three-Phase Parallel RLC Load  LConnTagsString=A|B|C  Configuration=Y (grounded)  NominalVoltage=22e3  Vabc=[1e3 1e3 1e3]  Vabcp=[1e3 1e3 1e3]  NominalFrequency=fNom  UnbalancedPower=off  ActivePower=5e6  InductivePower=0  CapacitivePower=0  Pabc=[10e3 9e3 11e3]  QLabc=[100 90 110]  QCabc=[100 90 110]  Pabcp=[10e3 9e3 11e3]  QLabcp=[100 90 110]  QCabcp=[100 90 110]  Measurements=None  LoadType=constant Z
  Bus Selector1 : BusSelector  OutputSignals="dq0 components.Stator voltage  vq (pu),dq0 components.Stator voltage  vd (pu),Mechanical.Rotor speed  wm  (pu),Mechanical.Rotor speed deviation  dw (pu),Output active power   Peo (pu),Output reactive power  Qeo (pu)"
  Bus 33 : powerlib/Measurements/Three-Phase V-I Measurement  VoltageMeasurement=phase-to-ground  SetLabelV=on  LabelV=V_bus_G4  Vpu=off  VpuLL=off  CurrentMeasurement=no  SetLabelI=on  LabelI=I_bus_G4  Ipu=off  Pbase=100e6  Vbase=16.5e3  OutputType=Complex  PhasorSimulation=off  PSBequivalent=0
  Excitation System1 : sps_avr/Excitation System  tr=20e-3  reg=[ 200, 0.02 ]  exc=[ 1, 0 .19]  tgr=[ 0, 0 ]  damp=[ 0.0012, 1 ]  sat=[ 0, 0 ]  lim=[ 0, 7.32, 0 ]  v0=[0.9972 1.7419]
      settings: SourceProductBaseCode=PS
  GT1_CB4 : Subsystem
  Ground : Ground
  HTG : powerlib/Machines/Hydraulic Turbine and Governor  sm="[ 10/3  0.07 ]"  gate="[  0.01  0.97518  -0.1  0.1 ]"  reg="[ Rp  1.163  0.105  0  0.01  ]"  hyd="[  0  2.67  ]"  dref=0  po=0.57
      settings: SourceProductBaseCode=PS
  Load Flow Bus : powerlib/Measurements/Load Flow Bus  LConnTagsString=a  Phases=single  Connectors=on one side  ID=Bus-33  Vbase=22000  Vref=0.9972  Vangle=0  VLF=0.9972  VLFb=1  VLFc=1  angleLF=-4.252  angleLFb=0  angleLFc=0
      settings: AttributesFormatString=%<ID>\n%<Vbase>V\n%<VLF>pu\n%<angleLF>deg.
  Machine 4 1000 MVA 22 kV : powerlib/Machines/Synchronous Machine pu Standard  PresetModel=No  MechanicalLoad=Mechanical power Pm  ShowDetailedParameters=on  RotorType=Round  Units=per unit standard parameters  MeasurementBus=off  NominalParameters="[ 1000E6  22000   fNom]"  Reactances1="[ 2.403 0.4 0.2 2.367 1.523 0.2 0.03  ]"  Reactances2=[ 0.995, 0.195, 0.155, 0.568, 0.143, 0.16 ]  dAxisTimeConstants=Open-circuit  qAxisTimeConstants=Open-circuit  TimeConstants1=[]  TimeConstants2=[5.69 0.03 1.5 0.04]  TimeConstants3=[]  TimeConstants4=[]  TimeConstants5=[ 9.2, 0.01, 0.01 ]  TimeConstants6=[]  TimeConstants7=[]  TimeConstants8=[]  StatorResistance=0.005  Mechanical=[ 3.117 0.02 20]  PolePairs=20  InitialConditions=[0 -47.2467 0.538718 0.538718 0.538718 -12.2371 -132.237 107.763 1.74187]  SetSaturation=off  Saturation=[0.6404,0.7127,0.8441,0.9214,0.9956,1.082,1.19,1.316,1.457;0.7,0.7698,0.8872,0.9466,0.9969,1.046,1.1,1.151,1.201]  LoadFlowParameters=[1 632000000 21938.4 0]  TsPowergui=0  TsBlock=-1  IterativeModel=Trapezoidal non iterative  IterativeDiscreteModel=Trapezoidal non iterative  BusType=PV  Pref=5.32e+008  Qref=0  Qmin=-500e6  Qmax=150e6  PLF=0  QLF=0
      settings: AttributesFormatString=\n\n
  Pref : Constant  Value=0.57
  Terminator5 : Terminator
  Transformer 4 1068.1 MVA 22 kV / 345 kV : powerlib/Elements/Three-Phase Transformer (Two Windings)  Winding1Connection=Delta (D1)  Winding2Connection=Yg  CoreType=Three single-phase transformers  SetSaturation=off  Hysteresis=off  DataFile='hysteresis'  SetInitialFlux=off  Measurements=None  UNITS=pu  NominalPower=[ 1068.1e6 fNom]  Winding1="[ 22e3 0.007*1068.1/100/2      0.0142*1068.1/100/2 ]"  Winding2="[ 1.07*345e3 0.007*1068.1/100/2      0.0142*1068.1/100/2]"  Rm=500  Lm=500  L0=0.5  Saturation="[ 0,0  ;  0.005,1.2  ;  1.0,1.4 ]"  InitialFluxes=[ 0.8 , -0.8 , 0.7 ]  BreakLoop=off  DiscreteSolver=Trapezoidal iterative  DataType=off  TransfoNumber=0
  Vref : Constant  Value=0.9972
  wref : Constant
  wref4 : Constant  Value=0
  A : PMIOPort  Side=Right
  B : PMIOPort  Port=2  Side=Right
  C : PMIOPort  Port=3  Side=Right
  tag scope: P_G4=global, Q_G4=global, V_G4=global, Wm_G4=global
  wires:
  [V_bus_G4] -> [V_G4]
  Bus Selector1/6 -> [Q_G4]  "<Output reactive power  Qeo (pu)>"
  Bus Selector1/5 -> [P_G4], HTG/4  "<Output active power   Peo (pu)>"
  Bus Selector1/4 -> HTG/5  "<Rotor speed deviation  dw (pu)>"
  Bus Selector1/3 -> [Wm_G4], HTG/3  "<Rotor speed  wm  (pu)>"
  Bus Selector1/2 -> Excitation System1/2  "<Stator voltage  vd (pu)>"
  Bus Selector1/1 -> Excitation System1/3  "<Stator voltage  vq (pu)>"
  Machine 4 1000 MVA 22 kV/1 -> Bus Selector1/1
  Excitation System1/1 -> Machine 4 1000 MVA 22 kV/2
  wref/1 -> HTG/1
  Pref/1 -> HTG/2
  Vref/1 -> Excitation System1/1
  HTG/2 -> Terminator5/1
  Ground/1 -> Excitation System1/4
  HTG/1 -> Machine 4 1000 MVA 22 kV/1
  connections:
  Machine 4 1000 MVA 22 kV/RConn3 -- Bus 33/LConn3
  Machine 4 1000 MVA 22 kV/RConn2 -- Bus 33/LConn2
  Machine 4 1000 MVA 22 kV/RConn1 -- Bus 33/LConn1
  5 MW/LConn3 -- Bus 33/RConn3 -- Transformer 4 1068.1 MVA 22 kV / 345 kV/LConn3
  5 MW/LConn2 -- Bus 33/RConn2 -- Transformer 4 1068.1 MVA 22 kV / 345 kV/LConn2
  5 MW/LConn1 -- Bus 33/RConn1 -- Load Flow Bus/LConn1 -- Transformer 4 1068.1 MVA 22 kV / 345 kV/LConn1
  GT1_CB4/LConn1 -- Transformer 4 1068.1 MVA 22 kV / 345 kV/RConn1
  GT1_CB4/LConn2 -- Transformer 4 1068.1 MVA 22 kV / 345 kV/RConn2
  GT1_CB4/LConn3 -- Transformer 4 1068.1 MVA 22 kV / 345 kV/RConn3
  C/RConn1 -- GT1_CB4/RConn3
  B/RConn1 -- GT1_CB4/RConn2
  A/RConn1 -- GT1_CB4/RConn1

== system model_FS_PSH_IEEE39/SS_EastSystem1/GT 5 ==
  5 MW : powerlib/Elements/Three-Phase Parallel RLC Load  LConnTagsString=A|B|C  Configuration=Y (grounded)  NominalVoltage=22e3  Vabc=[1e3 1e3 1e3]  Vabcp=[1e3 1e3 1e3]  NominalFrequency=fNom  UnbalancedPower=off  ActivePower=5e6  InductivePower=0  CapacitivePower=0  Pabc=[10e3 9e3 11e3]  QLabc=[100 90 110]  QCabc=[100 90 110]  Pabcp=[10e3 9e3 11e3]  QLabcp=[100 90 110]  QCabcp=[100 90 110]  Measurements=None  LoadType=constant Z
  Bus Selector1 : BusSelector  OutputSignals="dq0 components.Stator voltage  vq (pu),dq0 components.Stator voltage  vd (pu),Mechanical.Rotor speed  wm  (pu),Mechanical.Rotor speed deviation  dw (pu),Output active power   Peo (pu),Output reactive power  Qeo (pu)"
  Bus 34 : powerlib/Measurements/Three-Phase V-I Measurement  VoltageMeasurement=phase-to-ground  SetLabelV=on  LabelV=V_bus_G5  Vpu=off  VpuLL=off  CurrentMeasurement=no  SetLabelI=on  LabelI=I_bus_G5  Ipu=off  Pbase=100e6  Vbase=16.5e3  OutputType=Complex  PhasorSimulation=off  PSBequivalent=0
  Excitation System1 : sps_avr/Excitation System  tr=20e-3  reg=[ 200, 0.02 ]  exc=[ 1, 0 .19]  tgr=[ 0, 0 ]  damp=[ 0.0012, 1 ]  sat=[ 0, 0 ]  lim=[ 0, 7.32, 0 ]  v0=[1.0123 3.3412]
      settings: SourceProductBaseCode=PS
  GT1_CB6 : Subsystem
  Ground : Ground
  HTG : powerlib/Machines/Hydraulic Turbine and Governor  sm="[ 10/3  0.07 ]"  gate="[  0.01  0.97518  -0.1  0.1 ]"  reg="[  Rp  1.163  0.105  0  0.01  ]"  hyd="[  0  2.67  ]"  dref=0  po=0.709
      settings: SourceProductBaseCode=PS
  Load Flow Bus : powerlib/Measurements/Load Flow Bus  LConnTagsString=a  Phases=single  Connectors=on one side  ID=Bus-34  Vbase=22000  Vref=1.0123  Vangle=0  VLF=1.012  VLFb=1  VLFc=1  angleLF=-37.01  angleLFb=0  angleLFc=0
      settings: AttributesFormatString=%<ID>\n%<Vbase>V\n%<VLF>pu\n%<angleLF>deg.
  Machine 5 520 MVA 22 kV : powerlib/Machines/Synchronous Machine pu Standard  PresetModel=No  MechanicalLoad=Mechanical power Pm  ShowDetailedParameters=on  RotorType=Round  Units=per unit standard parameters  MeasurementBus=off  NominalParameters="[ 520E6  22000   fNom]"  Reactances1=[ 3.484 0.686 0.343 3.224 0.8632 0.343 0.054 ]  Reactances2=[ 0.995, 0.195, 0.155, 0.568, 0.143, 0.16 ]  dAxisTimeConstants=Open-circuit  qAxisTimeConstants=Open-circuit  TimeConstants1=[]  TimeConstants2=[5.4 0.03 0.44 0.04]  TimeConstants3=[]  TimeConstants4=[]  TimeConstants5=[ 9.2, 0.01, 0.01 ]  TimeConstants6=[]  TimeConstants7=[]  TimeConstants8=[]  StatorResistance=0  Mechanical=[ 5 0.02 20]  PolePairs=20  InitialConditions=[0 -74.2196 0.822255 0.822255 0.822255 -56.5136 -176.514 63.4864 3.34118]  SetSaturation=off  Saturation=[0.6404,0.7127,0.8441,0.9214,0.9956,1.082,1.19,1.316,1.457;0.7,0.7698,0.8872,0.9466,0.9969,1.046,1.1,1.151,1.201]  LoadFlowParameters=[1 508000000 22270.6 0]  TsPowergui=0  TsBlock=-1  IterativeModel=Trapezoidal non iterative  IterativeDiscreteModel=Trapezoidal non iterative  BusType=PV  Pref=4.08e+008  Qref=0  Qmin=-300e6  Qmax=200e6  PLF=0  QLF=0
      settings: AttributesFormatString=\n\n
  Pref : Constant  Value=0.709
  Terminator5 : Terminator
  Transformer 5 572 MVA 22 kV / 345 kV : powerlib/Elements/Three-Phase Transformer (Two Windings)  Winding1Connection=Delta (D1)  Winding2Connection=Yg  CoreType=Three single-phase transformers  SetSaturation=off  Hysteresis=off  DataFile='hysteresis'  SetInitialFlux=off  Measurements=None  UNITS=pu  NominalPower=[ 572e6 fNom]  Winding1="[ 22e3 0.009*572/100/2    0.018*572/100/2]"  Winding2="[ 1.009*345e3 0.009*572/100/2    0.018*572/100/2]"  Rm=500  Lm=500  L0=0.5  Saturation="[ 0,0  ;  0.005,1.2  ;  1.0,1.4 ]"  InitialFluxes=[ 0.8 , -0.8 , 0.7 ]  BreakLoop=off  DiscreteSolver=Trapezoidal iterative  DataType=off  TransfoNumber=0
  Vref : Constant  Value=1.0123
  wref : Constant
  A : PMIOPort  Side=Right
  B : PMIOPort  Port=2  Side=Right
  C : PMIOPort  Port=3  Side=Right
  tag scope: P_G5=global, Q_G5=global, V_G5=global, Wm_G5=global
  wires:
  Ground/1 -> Excitation System1/4
  HTG/2 -> Terminator5/1
  Vref/1 -> Excitation System1/1
  Pref/1 -> HTG/2
  wref/1 -> HTG/1
  HTG/1 -> Machine 5 520 MVA 22 kV/1
  Machine 5 520 MVA 22 kV/1 -> Bus Selector1/1
  Bus Selector1/1 -> Excitation System1/3  "<Stator voltage  vq (pu)>"
  Bus Selector1/2 -> Excitation System1/2  "<Stator voltage  vd (pu)>"
  Bus Selector1/3 -> HTG/3, [Wm_G5]  "<Rotor speed  wm  (pu)>"
  Bus Selector1/4 -> HTG/5  "<Rotor speed deviation  dw (pu)>"
  Bus Selector1/5 -> HTG/4, [P_G5]  "<Output active power   Peo (pu)>"
  Bus Selector1/6 -> [Q_G5]  "<Output reactive power  Qeo (pu)>"
  [V_bus_G5] -> [V_G5]
  Excitation System1/1 -> Machine 5 520 MVA 22 kV/2
  connections:
  Transformer 5 572 MVA 22 kV / 345 kV/LConn1 -- Load Flow Bus/LConn1 -- Bus 34/RConn1 -- 5 MW/LConn1
  Transformer 5 572 MVA 22 kV / 345 kV/LConn2 -- Bus 34/RConn2 -- 5 MW/LConn2
  Transformer 5 572 MVA 22 kV / 345 kV/LConn3 -- Bus 34/RConn3 -- 5 MW/LConn3
  Machine 5 520 MVA 22 kV/RConn1 -- Bus 34/LConn1
  Machine 5 520 MVA 22 kV/RConn2 -- Bus 34/LConn2
  Machine 5 520 MVA 22 kV/RConn3 -- Bus 34/LConn3
  GT1_CB6/LConn1 -- Transformer 5 572 MVA 22 kV / 345 kV/RConn1
  GT1_CB6/LConn2 -- Transformer 5 572 MVA 22 kV / 345 kV/RConn2
  GT1_CB6/LConn3 -- Transformer 5 572 MVA 22 kV / 345 kV/RConn3
  B/RConn1 -- GT1_CB6/RConn2
  A/RConn1 -- GT1_CB6/RConn1
  C/RConn1 -- GT1_CB6/RConn3

== system model_FS_PSH_IEEE39/SS_EastSystem1/Load 15 ==
  Bus_L15 : powerlib/Measurements/Three-Phase V-I Measurement  VoltageMeasurement=phase-to-ground  SetLabelV=off  LabelV=V_Bus_L15  Vpu=off  VpuLL=off  CurrentMeasurement=yes  SetLabelI=on  LabelI=I_L15  Ipu=off  Pbase=100e6  Vbase=230e3  OutputType=Complex  PhasorSimulation=off  PSBequivalent=0
  Terminator : Terminator
  Three-Phase Dynamic Load : powerlib/Elements/Three-Phase Dynamic Load  NominalVoltage=[345e3 fNom]  ActiveReactivePowers=[3.2e+08 1.53e+08]  PositiveSequence=[0.99604 18.5295]  ExternalControl=on  NpNq=[0 0]  TimeConstants="[0  0  0  0]"  MinimumVoltage=0.7  Tfilter=1e-4  LoadFlowParameters=[4,0,0,0,0]
      settings: SourceProductBaseCode=PS
  A : PMIOPort  Side=Left
  B : PMIOPort  Port=2  Side=Left
  C : PMIOPort  Port=3  Side=Left
  tag scope: V_L15=global
  wires:
  Three-Phase Dynamic Load/1 -> Terminator/1
  Bus_L15/1 -> [V_L15]
  [load15] -> Three-Phase Dynamic Load/1
  connections:
  C/RConn1 -- Bus_L15/LConn3
  Bus_L15/RConn3 -- Three-Phase Dynamic Load/LConn3
  Bus_L15/RConn2 -- Three-Phase Dynamic Load/LConn2
  A/RConn1 -- Bus_L15/LConn1
  B/RConn1 -- Bus_L15/LConn2
  Bus_L15/RConn1 -- Three-Phase Dynamic Load/LConn1

== system model_FS_PSH_IEEE39/SS_EastSystem1/Load 16 ==
  Bus_L16 : powerlib/Measurements/Three-Phase V-I Measurement  VoltageMeasurement=phase-to-ground  SetLabelV=off  LabelV=V_Bus_L16  Vpu=off  VpuLL=off  CurrentMeasurement=yes  SetLabelI=on  LabelI=I_L16  Ipu=off  Pbase=100e6  Vbase=230e3  OutputType=Complex  PhasorSimulation=off  PSBequivalent=0
  Terminator : Terminator
  Three-Phase Dynamic Load : powerlib/Elements/Three-Phase Dynamic Load  NominalVoltage=[345e3 fNom]  ActiveReactivePowers=[3.29e+08 3.23e+07]  PositiveSequence=[1.00736 19.2229]  ExternalControl=on  NpNq=[0 0]  TimeConstants="[0  0  0  0]"  MinimumVoltage=0.7  Tfilter=1e-4  LoadFlowParameters=[4,0,0,0,0]
      settings: SourceProductBaseCode=PS
  A : PMIOPort  Side=Left
  B : PMIOPort  Port=2  Side=Left
  C : PMIOPort  Port=3  Side=Left
  tag scope: V_L16=global
  wires:
  Three-Phase Dynamic Load/1 -> Terminator/1
  Bus_L16/1 -> [V_L16]
  [load16] -> Three-Phase Dynamic Load/1
  connections:
  Three-Phase Dynamic Load/LConn1 -- Bus_L16/RConn1
  C/RConn1 -- Bus_L16/LConn3
  B/RConn1 -- Bus_L16/LConn2
  A/RConn1 -- Bus_L16/LConn1
  Bus_L16/RConn2 -- Three-Phase Dynamic Load/LConn2
  Bus_L16/RConn3 -- Three-Phase Dynamic Load/LConn3

== system model_FS_PSH_IEEE39/SS_EastSystem1/Load 20 ==
  Bus_L20 : powerlib/Measurements/Three-Phase V-I Measurement  VoltageMeasurement=phase-to-ground  SetLabelV=off  LabelV=V_Bus_L20  Vpu=off  VpuLL=off  CurrentMeasurement=yes  SetLabelI=on  LabelI=I_L20  Ipu=off  Pbase=100e6  Vbase=230e3  OutputType=Complex  PhasorSimulation=off  PSBequivalent=0
  Snubber : powerlib/Elements/Three-Phase Series RLC Load  LConnTagsString=A|B|C  Configuration=Y (grounded)  NominalVoltage=345E3  Vabc=[1e3 1e3 1e3]  Vabcp=[1e3 1e3 1e3]  NominalFrequency=fNom  UnbalancedPower=off  ActivePower=1e6  InductivePower=0  CapacitivePower=1e7  Pabc=[10e3 9e3 11e3]  QLabc=[100 90 110]  QCabc=[100 90 110]  Pabcp=[10e3 9e3 11e3]  QLabcp=[100 90 110]  QCabcp=[100 90 110]  Measurements=None  LoadType=constant Z
  Terminator : Terminator
  Three-Phase Dynamic Load : powerlib/Elements/Three-Phase Dynamic Load  NominalVoltage=[345e3 fNom]  ActiveReactivePowers=[6.28e+08 1.03e+08]  PositiveSequence=[0.961329 -10.5466]  ExternalControl=on  NpNq=[0 0]  TimeConstants="[0  0  0  0]"  MinimumVoltage=0.7  Tfilter=1e-4  LoadFlowParameters=[4,0,0,0,0]
      settings: SourceProductBaseCode=PS
  A : PMIOPort  Side=Left
  B : PMIOPort  Port=2  Side=Left
  C : PMIOPort  Port=3  Side=Left
  tag scope: V_L20=global
  wires:
  Three-Phase Dynamic Load/1 -> Terminator/1
  Bus_L20/1 -> [V_L20]
  [load20] -> Three-Phase Dynamic Load/1
  connections:
  Bus_L20/RConn3 -- Snubber/LConn3 -- Three-Phase Dynamic Load/LConn3
  Bus_L20/RConn2 -- Snubber/LConn2 -- Three-Phase Dynamic Load/LConn2
  A/RConn1 -- Bus_L20/LConn1
  B/RConn1 -- Bus_L20/LConn2
  C/RConn1 -- Bus_L20/LConn3
  Bus_L20/RConn1 -- Snubber/LConn1 -- Three-Phase Dynamic Load/LConn1

== system model_FS_PSH_IEEE39/SS_EastSystem1/Machines Measurements ==
  Mux : Mux  Inputs=2
  Mux1 : Mux
  Mux2 : Mux
  Machines Measurements : Outport
  wires:
  Mux2/1 -> Mux/2
  Mux1/1 -> Mux/1
  Mux/1 -> Machines Measurements/1
  [Wm_G5] -> Mux2/4
  [Q_G5] -> Mux2/3
  [P_G5] -> Mux2/2
  [V_G5] -> Mux2/1
  [Wm_G4] -> Mux1/4
  [Q_G4] -> Mux1/3
  [P_G4] -> Mux1/2
  [V_G4] -> Mux1/1

== system model_FS_PSH_IEEE39/SS_EastSystem2/Buses current_E ==
  Mux3 : Mux
  current : Outport
  wires:
  Mux3/1 -> current/1
  [I_L21] -> Mux3/1
  [I_bus_22] -> Mux3/2
  [I_L23] -> Mux3/3
  [I_L24] -> Mux3/4

== system model_FS_PSH_IEEE39/SS_EastSystem2/Buses voltages_E ==
  Mux3 : Mux
  Voltages : Outport
  wires:
  [V_L24] -> Mux3/4
  [V_L23] -> Mux3/3
  [V_bus_22] -> Mux3/2
  [V_L21] -> Mux3/1
  Mux3/1 -> Voltages/1
